simulink model "P5_0_Simple_Model"  (R2025b)
settings: Solver=VariableStepAuto  StartTime=0.0  StopTime=10.0  RelTol=1e-3
settings Model: Creator=tongx  LastModifiedBy=tongx

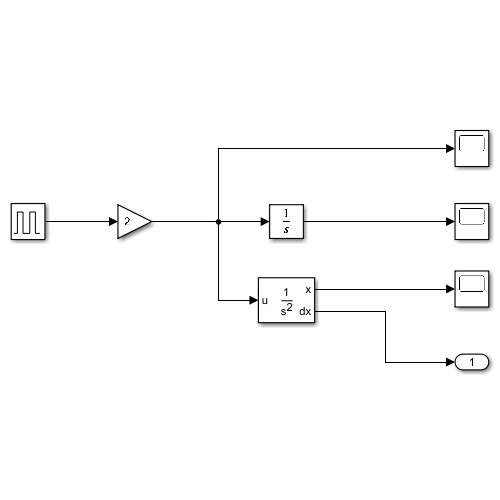
[thumbnail: Simulink's stored preview of the top-level diagram]
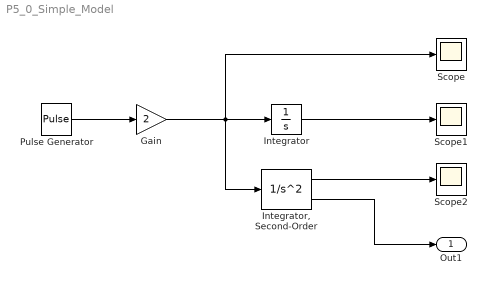
== system P5_0_Simple_Model ==
  Gain : Gain  Gain=2
  Integrator : Integrator
  "Integrator, Second-Order" : SecondOrderIntegrator
  Pulse Generator : DiscretePulseGenerator  PulseType=Time based  Period=1  PulseWidth=5
  Scope : Scope
      settings: ActiveDisplayYMinimum=-13.666312025820153  ActiveDisplayYMaximum=14.870304658327054
  Scope1 : Scope
      settings: ActiveDisplayYMinimum=-0.12500000000000008  ActiveDisplayYMaximum=1.1250000000000009
  Scope2 : Scope
      settings: ActiveDisplayYMinimum=-0.68437499999999929  ActiveDisplayYMaximum=6.1593749999999945  DataLoggingVariableName=ScopeData2
  Out1 : Outport
  wires:
  Pulse Generator/1 -> Gain/1
  Gain/1 -> Scope/1, "Integrator, Second-Order"/1, Integrator/1
  Integrator/1 -> Scope1/1
  "Integrator, Second-Order"/1 -> Scope2/1
  "Integrator, Second-Order"/2 -> Out1/1
